simulink model "sfbk"  (R2015a)
settings: Solver=ode4  StartTime=0.0  StopTime=1  FixedStep=0.01  RelTol=1e-3
values from neighbouring files (symbols this model uses):
  A = [ 0 1 1 ... (first row only)    [controllable.m]    (also in poleplace.m = [ -3 1; poleplace_acker.m = [ -3 1; poleplace_ctrb.m = [ -3 1; poleplace_place.m = [ 0 1 0 0)
  B = [0 1 ... (first row only)    [controllable.m]    (also in poleplace.m = [2 0]'; poleplace_acker.m = [2 0]'; poleplace_ctrb.m = [2 0]'; poleplace_place.m = [ 0 0)
  C = eye(2)    [poleplace_acker.m]
  D = zeros(2,1)    [poleplace_acker.m]
  K = subs([k1 k2],{p1 p2},{-8+4j, -8-4j})    [poleplace.m]    (also in poleplace_acker.m = -acker(A,B,p); poleplace_ctrb.m = Kc*Tc; poleplace_place.m = -place(A,B,p))
  x0 = [1 0]'    [poleplace_acker.m]
settings Model: Creator=shohei  LastModifiedBy=shohei

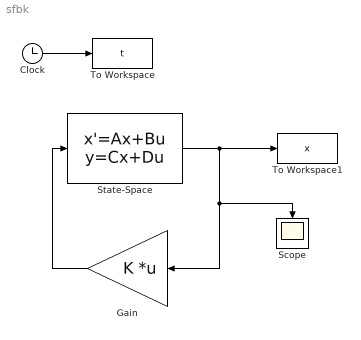
== system sfbk ==
  Clock : Clock
  Gain : Gain  Gain=K  Multiplication=Matrix(K*u)
  Scope : Scope
  State-Space : StateSpace  A=A  B=B  C=C  D=D  X0=x0
  To Workspace : ToWorkspace  VariableName=t  SampleTime=-1
  To Workspace1 : ToWorkspace  VariableName=x  SampleTime=-1
  wires:
  Clock/1 -> To Workspace/1
  Gain/1 -> State-Space/1
  State-Space/1 -> Gain/1, Scope/1, To Workspace1/1
